simulink model "problem5"  (R2020b)
settings: Solver=VariableStepAuto  StartTime=0.0  StopTime=10.0  RelTol=1e-3
model workspace (MAT data in the model file):
  C = 10
  R = 10
settings Model: Creator=admin  LastModifiedBy=admin

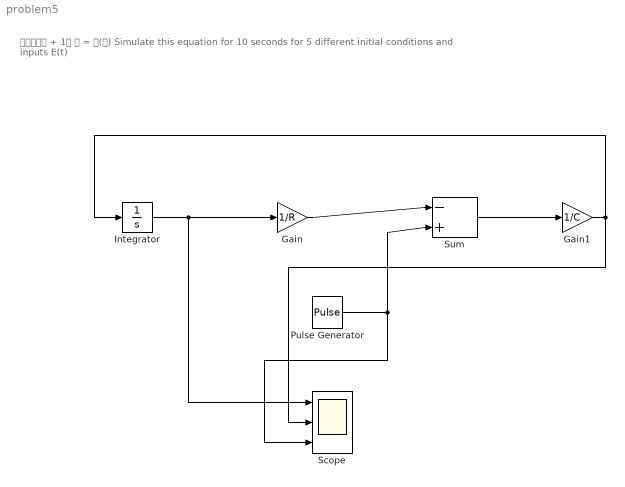
== system problem5 ==
  note: 𝑅𝑑𝑄𝑑𝑡 + 1𝐶 𝑄 = 𝐸(𝑡)
      | Simulate this equation for 10 seconds for 5 different initial conditions and inputs E(t)
  Gain : Gain  Gain=1/R
  Gain1 : Gain  Gain=1/C
  Integrator : Integrator  InitialCondition=1
  Pulse Generator : DiscretePulseGenerator  PulseType=Time based  Period=10  PulseWidth=5
  Scope : Scope  NumInputPorts=3
  Sum : Sum  Inputs=|-+
  wires:
  Integrator/1 -> Scope/1, Gain/1
  Gain/1 -> Sum/1
  Sum/1 -> Gain1/1
  Gain1/1 -> Scope/2, Integrator/1
  Pulse Generator/1 -> Scope/3, Sum/2
